simulink model "Noeud_HDL"  (R2017a)
settings: Solver=VariableStepAuto  StartTime=0.0  StopTime=1  RelTol=1e-3
libraries: commrandsrc3 x1
settings Model: SimulationMode=accelerator  Creator=floriant  LastModifiedBy=floriant
settings OptimizationCC: BlockReduction=off  ConditionallyExecuteInputs=off

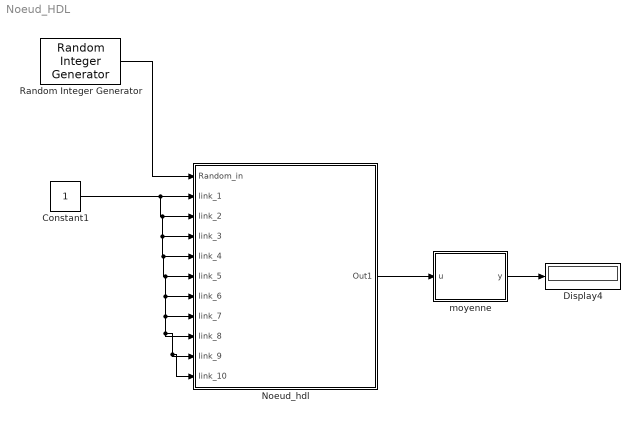
== system Noeud_HDL ==
  Constant1 : Constant  OutDataTypeStr=boolean  SampleTime=-1
  Display4 : Display
  Noeud_hdl : Subsystem
  Random Integer Generator : commrandsrc3/Random Integer Generator  SetSize=1000  SeedSource=Auto  Seed=0  SampleTime=1e-6  SamplesPerFrame=1  OutputDataType=uint16  SimulateUsing=Interpreted execution
  moyenne : MATLAB Function  TreatAsAtomicUnit=on
  wires:
  Random Integer Generator/1 -> Noeud_hdl/1(Random_in)
  Noeud_hdl/1(Out1) -> moyenne/1(u)
  moyenne/1(y) -> Display4/1
  Constant1/1 -> Noeud_hdl/11(link_10), Noeud_hdl/10(link_9), Noeud_hdl/9(link_8), Noeud_hdl/8(link_7), Noeud_hdl/7(link_6), Noeud_hdl/6(link_5), Noeud_hdl/5(link_4), Noeud_hdl/4(link_3), Noeud_hdl/3(link_2), Noeud_hdl/2(link_1)

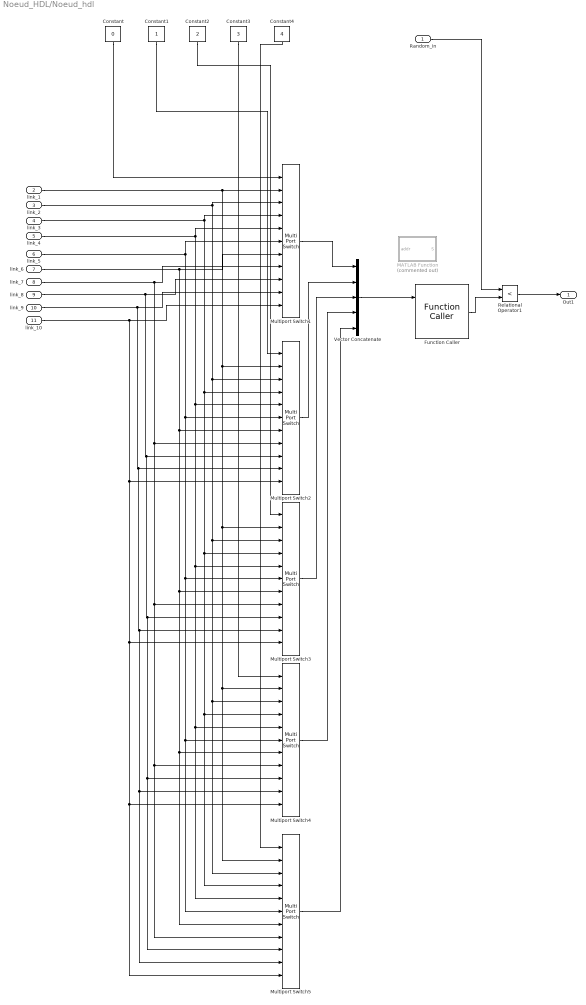
== system Noeud_HDL/Noeud_hdl ==
  Random_in : Inport  OutDataTypeStr=uint16
  link_1 : Inport  Port=2  OutDataTypeStr=boolean
  link_2 : Inport  Port=3  OutDataTypeStr=boolean
  link_3 : Inport  Port=4  OutDataTypeStr=boolean
  link_4 : Inport  Port=5  OutDataTypeStr=boolean
  link_5 : Inport  Port=6  OutDataTypeStr=boolean
  link_6 : Inport  Port=7  OutDataTypeStr=boolean
  link_7 : Inport  Port=8  OutDataTypeStr=boolean
  link_8 : Inport  Port=9  OutDataTypeStr=boolean
  link_9 : Inport  Port=10  OutDataTypeStr=boolean
  link_10 : Inport  Port=11  OutDataTypeStr=boolean
  Constant : Constant  Value=0  OutDataTypeStr=uint8  SampleTime=-1
  Constant1 : Constant  OutDataTypeStr=uint8  SampleTime=-1
  Constant2 : Constant  Value=2  OutDataTypeStr=uint8  SampleTime=-1
  Constant3 : Constant  Value=3  OutDataTypeStr=uint8  SampleTime=-1
  Constant4 : Constant  Value=4  OutDataTypeStr=uint8  SampleTime=-1
  Function Caller : FunctionCaller  FunctionPrototype=S = Memory(addr,Node1)
  MATLAB Function : MATLAB Function  Commented=on  TreatAsAtomicUnit=on
  Multiport Switch{1..5} (5 alike) : MultiPortSwitch  DataPortOrder=Zero-based contiguous  Inputs=10
  Relational Operator1 : RelationalOperator  Operator=<  OutDataTypeStr=boolean  RndMeth=Nearest  InputSameDT=on
  Vector Concatenate : Concatenate  NumInputs=5
  Out1 : Outport  OutDataTypeStr=boolean
  wires:
  Multiport Switch2/1 -> Vector Concatenate/2
  Random_in/1 -> Relational Operator1/1
  Multiport Switch5/1 -> Vector Concatenate/5
  link_4/1 -> Multiport Switch1/5, Multiport Switch5/5, Multiport Switch4/5, Multiport Switch3/5, Multiport Switch2/5
  Constant1/1 -> Multiport Switch2/1
  Constant2/1 -> Multiport Switch3/1
  Relational Operator1/1 -> Out1/1
  link_1/1 -> Multiport Switch5/2, Multiport Switch4/2, Multiport Switch3/2, Multiport Switch2/2, Multiport Switch1/2
  Constant3/1 -> Multiport Switch4/1
  link_8/1 -> Multiport Switch5/9, Multiport Switch4/9, Multiport Switch3/9, Multiport Switch2/9, Multiport Switch1/9
  link_9/1 -> Multiport Switch5/10, Multiport Switch4/10, Multiport Switch3/10, Multiport Switch2/10, Multiport Switch1/10
  Constant4/1 -> Multiport Switch5/1
  link_10/1 -> Multiport Switch5/11, Multiport Switch4/11, Multiport Switch3/11, Multiport Switch2/11, Multiport Switch1/11
  link_3/1 -> Multiport Switch5/4, Multiport Switch4/4, Multiport Switch3/4, Multiport Switch2/4, Multiport Switch1/4
  link_2/1 -> Multiport Switch5/3, Multiport Switch4/3, Multiport Switch3/3, Multiport Switch2/3, Multiport Switch1/3
  link_7/1 -> Multiport Switch5/8, Multiport Switch4/8, Multiport Switch3/8, Multiport Switch2/8, Multiport Switch1/8
  Multiport Switch1/1 -> Vector Concatenate/1
  link_6/1 -> Multiport Switch3/7, Multiport Switch5/7, Multiport Switch4/7, Multiport Switch2/7, Multiport Switch1/7
  link_5/1 -> Multiport Switch1/6, Multiport Switch5/6, Multiport Switch4/6, Multiport Switch3/6, Multiport Switch2/6
  Constant/1 -> Multiport Switch1/1
  Multiport Switch4/1 -> Vector Concatenate/4
  Multiport Switch3/1 -> Vector Concatenate/3
  Vector Concatenate/1 -> Function Caller/1
  Function Caller/1 -> Relational Operator1/2

== matlab function Noeud_HDL/moyenne ==
  data: u input; y output
function y = fcn(u)
persistent nb_one total
if isempty(nb_one)
    nb_one=0;
end
if isempty(total)
    total=0;
end
if u==1
    nb_one = nb_one+1;
end
total = total +1;

y=nb_one/total;

== matlab function Noeud_HDL/Noeud_hdl/MATLAB Function ==
  data: addr input; S output
function S = fcn(addr)
MEM =[950;290;940;1];
S=uint16(MEM(addr+1));
